simulink model "model1"  (R2017b)
settings: Solver=VariableStepAuto  StartTime=0.0  StopTime=10.0  RelTol=1e-3
settings Model: Creator=ladislav  LastModifiedBy=ladislav

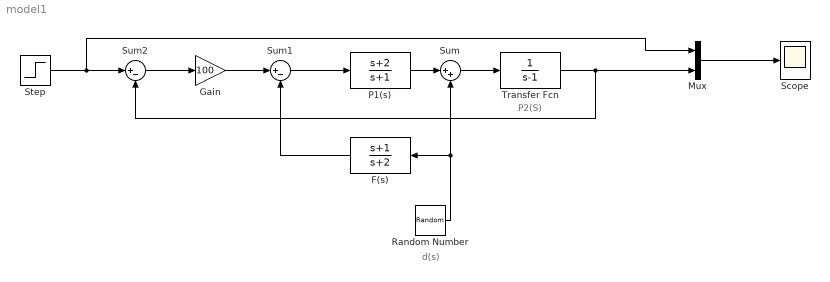
== system model1 ==
  note: d(s)
  note: P2(S)
  F(s) : TransferFcn  Numerator=[1 1]  Denominator=[1 2]
  Gain : Gain  Gain=100
  Mux : Mux  Inputs=2
  P1(s) : TransferFcn  Numerator=[1 2]  Denominator=[1 1]
  Random Number : RandomNumber  SampleTime=0.1
  "Scope " : Scope
  "Step " : Step  SampleTime=0
  Sum : Sum  Inputs=|++
  Sum1 : Sum  Inputs=|+-
  Sum2 : Sum  Inputs=|+-
  Transfer Fcn : TransferFcn  Denominator=[1 -1]
  wires:
  P1(s)/1 -> Sum/1
  Sum/1 -> Transfer Fcn/1
  Sum1/1 -> P1(s)/1
  Transfer Fcn/1 -> Mux/2, Sum2/2
  F(s)/1 -> Sum1/2
  Random Number/1 -> Sum/2, F(s)/1
  "Step "/1 -> Mux/1, Sum2/1
  Mux/1 -> "Scope "/1
  Sum2/1 -> Gain/1
  Gain/1 -> Sum1/1
